simulink library "sm_car_scene_crg_slope"  (R2018b)
settings: Solver=VariableStepAuto  StartTime=0.0  StopTime=10.0  RelTol=1e-3
undefined symbols (not defined in the file or in its folder): Scene
libraries: sm_car_lib x1
Description:
  | Scene of Simscape Vehicle Templates Library
  | 
  | Copyright 2018-2020 The MathWorks, Inc.
settings Model: Creator=smiller  LastModifiedBy=smiller

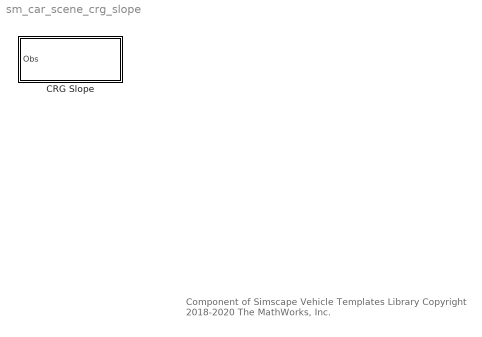
== system sm_car_scene_crg_slope ==
  note: Component of Simscape Vehicle Templates Library
      | Copyright 2018-2020 The MathWorks, Inc.
  CRG Slope : Subsystem  mask{geometry=Scene.CRG_Slope.Geometry}
      mask prompts: geometry "Geometry (structure)"

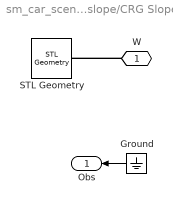
== system sm_car_scene_crg_slope/CRG Slope ==
  Ground : Ground
  STL Geometry : sm_car_lib/Environment/STL Geometry  stl_file=geometry.filename  stl_units=geometry.fileunits  stl_clr=geometry.clr  stl_opc=geometry.opc  stl_x=geometry.x  stl_y=geometry.y  stl_z=geometry.z  stl_yaw=geometry.yaw  stl_pitch=geometry.pitch  stl_roll=geometry.roll
  W : PMIOPort  Side=Left
  Obs : Outport
  wires:
  Ground/1 -> Obs/1
  connections:
  W/RConn1 -- STL Geometry/RConn1
